simulink model "DC_Charger"  (R2024b)
settings: Solver=ode23t  StartTime=0.0  StopTime=inf  FixedStep=1e-6  MaxStep=1/(5*inverter.SwitchFrequency)  RelTol=1e-3  AbsTol=1e-3
undefined symbols (not defined in the file or in its folder): battery, inverter, rectifier
libraries: nesl_utility x38, fl_lib x26, ee_lib x14, batteryecm_lib x3, eePwmGenerator x2, eeTransforms x2, eeSinusoidalMeasurement x1, slpidlib x1, eePwmGeneratorThreeLevel x1, eePwmGeneratorTwoLevel x1, simulink_extras x1
(part 3 of 3)

== system DC_Charger/EV Battery/i ==
  Current Sensor : fl_lib/Electrical/Electrical Sensors/Current Sensor
  PS-Simulink Converter1 : nesl_utility/PS-Simulink Converter  PhysicalDomain=network_engine_domain  SubClassName=ps_output  LeftPortType=input  RightPortType=output  PseudoPeriodic=off  Frequencies=[]  VectorFormat=1-D array  Unit=1  AffineConversion=off
  Rate Transition : RateTransition  OutPortSampleTime=1/(10*inverter.SwitchFrequency)
  + : PMIOPort  Side=Left
  - : PMIOPort  Port=2  Side=Right
  I : Outport
  wires:
  Rate Transition/1 -> I/1
  PS-Simulink Converter1/1 -> Rate Transition/1
  connections:
  Current Sensor/RConn1 -- PS-Simulink Converter1/LConn1
  Current Sensor/RConn2 -- -/RConn1
  Current Sensor/LConn1 -- +/RConn1

== system DC_Charger/EV Battery/v ==
  PS-Simulink Converter : nesl_utility/PS-Simulink Converter  PhysicalDomain=network_engine_domain  SubClassName=ps_output  LeftPortType=input  RightPortType=output  PseudoPeriodic=off  Frequencies=[]  VectorFormat=1-D array  Unit=1  AffineConversion=off
  Rate Transition : RateTransition  OutPortSampleTime=1/(10*inverter.SwitchFrequency)
  Voltage Sensor : fl_lib/Electrical/Electrical Sensors/Voltage Sensor
  + : PMIOPort  Side=Right
  - : PMIOPort  Port=2  Side=Left
  V : Outport
  wires:
  PS-Simulink Converter/1 -> Rate Transition/1
  Rate Transition/1 -> V/1
  connections:
  +/RConn1 -- Voltage Sensor/LConn1
  -/RConn1 -- Voltage Sensor/RConn2
  Voltage Sensor/RConn1 -- PS-Simulink Converter/LConn1

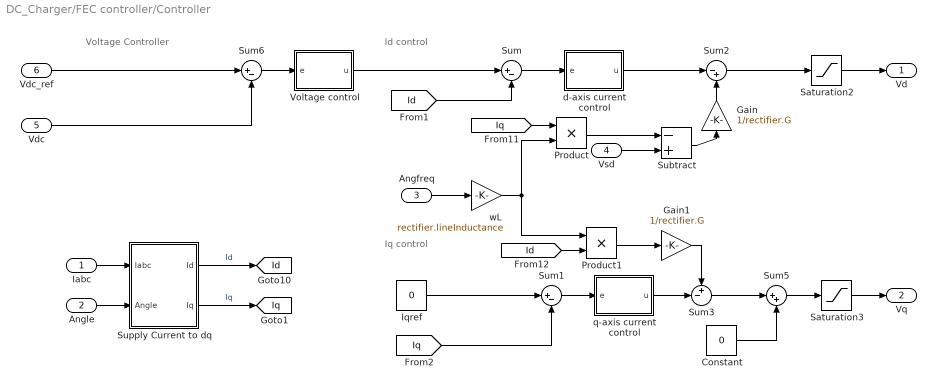
== system DC_Charger/FEC controller/Controller ==
  note: Id control
  note: Voltage Controller
  note: Iq control
  Iabc : Inport
  Angle : Inport  Port=2
  Angfreq : Inport  Port=3
  Vsd : Inport  Port=4
  Vdc : Inport  Port=5
  Vdc_ref : Inport  Port=6
  Constant : Constant  Value=0
  Gain : Gain  Gain=1/rectifier.G
  Gain1 : Gain  Gain=1/rectifier.G
  Iqref : Constant  Value=0
  Product : Product
  Product1 : Product
  Saturation2 : Saturate  UpperLimit=4  LowerLimit=-3
  Saturation3 : Saturate  UpperLimit=1  LowerLimit=-1
  Subtract : Sum  Inputs=-+
  Sum : Sum  Inputs=|+-
  Sum1 : Sum  Inputs=|+-
  Sum2 : Sum  Inputs=|-+
  Sum3 : Sum  Inputs=+-|
  Sum5 : Sum  Inputs=|++
  Sum6 : Sum  Inputs=|+-
  Supply Current to dq : Subsystem
  Voltage control : Subsystem
  d-axis current control : Subsystem
  q-axis current control : Subsystem
  wL : Gain  Gain=rectifier.lineInductance
  Vd : Outport  VectorParamsAs1DForOutWhenUnconnected=off
  Vq : Outport  Port=2  VectorParamsAs1DForOutWhenUnconnected=off
  tag scope: Id=global, Iq=global
  wires:
  Sum1/1 -> q-axis current control/1(e)
  wL/1 -> Product/2, Product1/1
  [Id] -> Product1/2
  [Iq] -> Product/1
  Sum3/1 -> Sum5/1
  Sum2/1 -> Saturation2/1
  Sum5/1 -> Saturation3/1
  Angfreq/1 -> wL/1
  Constant/1 -> Sum5/2
  Vdc/1 -> Sum6/2
  Sum/1 -> d-axis current control/1(e)
  [Id] -> Sum/2
  d-axis current control/1(u) -> Sum2/1
  q-axis current control/1(u) -> Sum3/2
  Supply Current to dq/1(Id) -> [Id]  "Id"
  Supply Current to dq/2(Iq) -> [Iq]  "Iq"
  Sum6/1 -> Voltage control/1(e)
  Saturation3/1 -> Vq/1
  Saturation2/1 -> Vd/1
  Iqref/1 -> Sum1/1
  [Iq] -> Sum1/2
  Voltage control/1(u) -> Sum/1
  Vdc_ref/1 -> Sum6/1
  Product1/1 -> Gain1/1
  Product/1 -> Subtract/1
  Vsd/1 -> Subtract/2
  Subtract/1 -> Gain/1
  Gain/1 -> Sum2/2
  Gain1/1 -> Sum3/1
  Iabc/1 -> Supply Current to dq/1(Iabc)
  Angle/1 -> Supply Current to dq/2(Angle)

== system DC_Charger/FEC controller/Modulation Signal ==
  Vd : Inport
  Vq : Inport  Port=2
  Angle : Inport  Port=3
  Constant : Constant  Value=0
  Gain : Gain  Gain=2/3
  Inverse Park Transform : eeTransforms/Inverse Park Transform  AxisAlignment=D-axis  PowerInvariant=off
  Mux1 : Mux  Inputs=3
  Saturation2 : Saturate  UpperLimit=1  LowerLimit=-1
  mabc : Outport  VectorParamsAs1DForOutWhenUnconnected=off
  wires:
  Gain/1 -> Saturation2/1
  Mux1/1 -> Inverse Park Transform/1
  Inverse Park Transform/1 -> Gain/1
  Constant/1 -> Mux1/3
  Vd/1 -> Mux1/1
  Vq/1 -> Mux1/2
  Angle/1 -> Inverse Park Transform/2
  Saturation2/1 -> mabc/1

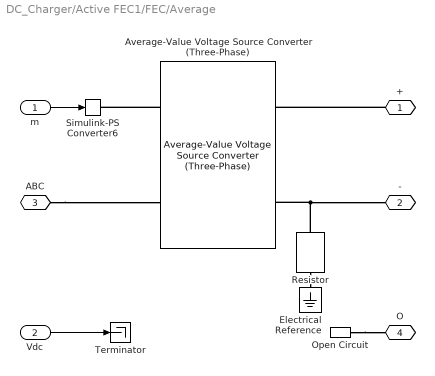
== system DC_Charger/Active FEC1/FEC/Average ==
  m : Inport
  Vdc : Inport  Port=2
  Average-Value Voltage Source Converter (Three-Phase) : ee_lib/Semiconductors & Converters/Converters/Average-Value Voltage Source Converter (Three-Phase)  port_option=ee.enum.threePhasePort.composite  frequency_option=ee.enum.converters.frequency.variable  input_option=ee.enum.converters.inputOption.ModWave  FRated=60 Hz  losses_parameterization=ee.enum.converters.losses.fixed  Pfixed=1 W  ks=0.01  kc1=1.7 V  kc2=0.01 Ohm  Ploss_vect=[100, 800, 1870, 3250, 4900] W  Irms_vect=[10, 100, 200, 300, 400] A  Vdc_nom=300 V  thermal_mass=30000 J/K  temperature_specify=off  temperature_priority=High  temperature=298.15 K  temperature_nominal_specify=off  temperature_nominal_value=1  temperature_nominal_unit=K
      settings: InternalSimscapePortConfiguration="{\"Bottom\":[],\"Left\":[{\"id\":\"ModWave\",\"label\":\"ModWave\",\"type\":\"input\"},{\"id\":\"N\",\"label\":\"~\",\"type\":\"foundation.electrical.three_phase\"}],\"Right\":[{\"id\":\"p\",\"label\":\"+\",\"type\":\"foundation.electrical.electrical\"},{\"id\":\"n\",\"label\":\"-\",\"type\":\"foundation.electrical.electrical\"}],\"Top\":[]}"
  Electrical Reference : fl_lib/Electrical/Electrical Elements/Electrical Reference
  Open Circuit : fl_lib/Electrical/Electrical Elements/Open Circuit  v_specify=off  v_priority=None  v=0 V  v_nominal_specify=off  v_nominal_value=1  v_nominal_unit=V
  Resistor : fl_lib/Electrical/Electrical Elements/Resistor  R=1e6 Ohm  i_specify=off  i_priority=None  i=0 A  i_nominal_specify=off  i_nominal_value=1  i_nominal_unit=A  v_specify=off  v_priority=None  v=0 V  v_nominal_specify=off  v_nominal_value=1  v_nominal_unit=V
  Simulink-PS Converter6 : nesl_utility/Simulink-PS Converter  PhysicalDomain=network_engine_domain  SubClassName=ps_input  LeftPortType=input  RightPortType=output  PseudoPeriodic=off  Frequencies=[]  NoiseDistribution=none  NoiseParameters=[]  Unit=1  AffineConversion=off  FilteringAndDerivatives=provide  SimscapeFilterOrder=1  InputFilterTimeConstant=0.001  UdotUserProvided=0
  Terminator : Terminator
  + : PMIOPort  Side=Right
  - : PMIOPort  Port=2  Side=Right
  ABC : PMIOPort  Port=3  Side=Left
  O : PMIOPort  Port=4  Side=Right
  wires:
  m/1 -> Simulink-PS Converter6/1
  Vdc/1 -> Terminator/1
  connections:
  Open Circuit/LConn1 -- O/RConn1
  Average-Value Voltage Source Converter (Three-Phase)/LConn1 -- Simulink-PS Converter6/RConn1
  ABC/RConn1 -- Average-Value Voltage Source Converter (Three-Phase)/LConn2
  +/RConn1 -- Average-Value Voltage Source Converter (Three-Phase)/RConn1
  Resistor/LConn1 -- Average-Value Voltage Source Converter (Three-Phase)/RConn2 -- -/RConn1
  Resistor/RConn1 -- Electrical Reference/LConn1

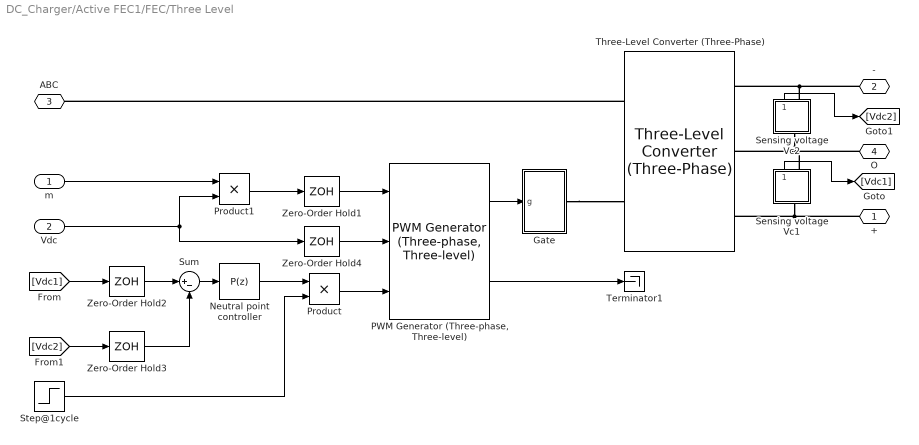
== system DC_Charger/Active FEC1/FEC/Three Level ==
  m : Inport
  Vdc : Inport  Port=2
  Gate : Subsystem
  Neutral point controller : slpidlib/PID Controller  Controller=P  Form=Parallel  TimeDomain=Discrete-time  UseExternalTs=off  SampleTime=-1  IntegratorMethod=Forward Euler  FilterMethod=Forward Euler  ControllerParametersSource=internal  P=0.001  I=80/2  UseKiTs=off  D=0  UseExternalDerivativeSource=off  N=100  UseFilter=on  TunerSelectOption=Transfer Function Based (PID Tuner App)  ZeroCross=off  InitialConditionSource=internal  InitialConditionForIntegrator=0  InitialConditionForFilter=0  DifferentiatorICPrevScaledInput=0  ExternalReset=none  TrackingMode=off  Kt=1  LimitOutput=on  SatLimitsSource=internal  UpperSaturationLimit=1  LowerSaturationLimit=-1  LinearizeAsGain=on  AntiWindupMode=back-calculation  Kb=1000  LimitIntegrator=off  UpperIntegratorSaturationLimit=inf  LowerIntegratorSaturationLimit=-inf  POutMin=[]  POutMax=[]  IOutMin=[]  IOutMax=[]  DOutMin=[]  DOutMax=[]  NOutMin=[]  NOutMax=[]  SumOutMin=[]  SumOutMax=[]  SaturationOutMin=[]  SaturationOutMax=[]  PParamMin=[]  PParamMax=[]  IParamMin=[]  IParamMax=[]  DParamMin=[]  DParamMax=[]  NParamMin=[]  NParamMax=[]  KbParamMin=[]  KbParamMax=[]  KtParamMin=[]  KtParamMax=[]  KbOutMin=[]  KbOutMax=[]  KtOutMin=[]  KtOutMax=[]  IntegratorOutMin=[]  IntegratorOutMax=[]  FilterOutMin=[]  FilterOutMax=[]  SumI1OutMin=[]  SumI1OutMax=[]  SumI2OutMin=[]  SumI2OutMax=[]  SumI3OutMin=[]  SumI3OutMax=[]  SumI4OutMin=[]  SumI4OutMax=[]  SumDOutMin=[]  SumDOutMax=[]  DifferentiatorOutMin=[]  DifferentiatorOutMax=[]  FilterDiffOutCoefMin=[]  FilterDiffOutCoefMax=[]  ReciprocalOutMin=[]  ReciprocalOutMax=[]  SumDenOutMin=[]  SumDenOutMax=[]  SumNumOutMin=[]  SumNumOutMax=[]  DivideOutMin=[]  DivideOutMax=[]  UdiffTsProdOutMin=[]  UdiffTsProdOutMax=[]  NTsProdOutMin=[]  NTsProdOutMax=[]  UintegralTsProdOutMin=[]  UintegralTsProdOutMax=[]  UngainTsProdOutMin=[]  UngainTsProdOutMax=[]  ClampingZeroOutDataTypeStr=Inherit: Inherit via back propagation  ClampingZeroOutMin=[]  ClampingZeroOutMax=[]  FilterDenConstantOutDataTypeStr=Inherit: Inherit via back propagation  FilterDenConstantOutMin=[]  FilterDenConstantOutMax=[]  PCopyOutDataTypeStr=Inherit: Inherit via back propagation  PCopyOutMin=[]  PCopyOutMax=[]  NCopyOutDataTypeStr=Inherit: Inherit via back propagation  NCopyOutMin=[]  NCopyOutMax=[]  IntegratorContinuousStateAttributes=''  IntegratorStateMustResolveToSignalObject=off  IntegratorRTWStateStorageClass=Auto  FilterContinuousStateAttributes=''  FilterStateMustResolveToSignalObject=off  FilterRTWStateStorageClass=Auto  ParallelPVariant=InternalParameters  IdealPVariant=Disabled  IVariant=Disabled  DVariant=Disabled  IntegratorVariant=Disabled  SatVariant=Enabled  AWVariant=Disabled  PCopyVariant=Disabled  TRVariant=Disabled  FdbkBlocksVariant=Forward  IdealPFdbkVariant=Disabled  SatFdbkVariant=Disabled  DerivativeFilterVariant=Disabled  NVariant=Disabled  NCopyVariant=Disabled_SignalSpec  FilterICVariant=Disabled  IntegratorICVariant=Disabled  ExternalResetVariant=Disabled  TRSumVariant=Passthrough  SumFdbkVariant=Disabled  SumVariant=Passthrough_P  TsampFilterVariant=InternalTs  TsampNgainVariant=Passthrough  TsampIntegralVariant=Disabled_SignalSpec  ExternalSaturationOutDataTypeStr=Inherit: Same as second input  DerivativeSourceVariant=Disabled  PreIntVariant=InternalPreInt
  "PWM Generator (Three-phase, Three-level)" : eePwmGeneratorThreeLevel/PWM Generator (Three-phase, Three-level)  CPWMMode=SPWM: sinusoidal PWM  fsw=rectifier.SwitchFrequency  Ts=1/(10*rectifier.SwitchFrequency)
      settings: SamplingMode=Natural
  Product : Product
  Product1 : Product
  Sensing voltage Vc1 : Subsystem
      mask Display: disp('Vdc1')
  Sensing voltage Vc2 : Subsystem
      mask Display: disp('Vdc2')
  Step@1cycle : Step  Time=1/rectifier.SystemFrequency  SampleTime=1/(10*rectifier.SwitchFrequency)
  Sum : Sum  Inputs=|+-
  Terminator1 : Terminator
  Three-Level Converter (Three-Phase) : ee_lib/Semiconductors & Converters/Converters/Three-Level Converter (Three-Phase)  port_option=ee.enum.threePhasePort.composite  device_type=2  Vf=0.8 V  Ron=0.001 Ohm  Rds=0.001 Ohm  Goff=1e-6 1/Ohm  Vth=0.2 V  Vgt=1 V  Vgt_off=-1 V  Ih=1 A  K=0  diode_param=2  diode_Vf=0.8 V  diode_Ron=0.001 Ohm  diode_Goff=1e-5 1/Ohm  diode_C=50 nF  diode_iRM=-235 A  diode_iF=300 A  diode_idot=-50 A/us  diode_trr_param=1  diode_trr_factor=3  diode_trr=15 us  diode_Qrr=1500 s*uA  snubber_type=0  Cs=1e-7 F  Rs=0.1 Ohm
      settings: InternalSimscapePortConfiguration="{\"Bottom\":[],\"Left\":[{\"id\":\"G\",\"label\":\"G\",\"type\":\"foundation.electrical.twenty_four_phase\"},{\"id\":\"N\",\"label\":\"~\",\"type\":\"foundation.electrical.three_phase\"}],\"Right\":[{\"id\":\"p\",\"label\":\"+\",\"type\":\"foundation.electrical.electrical\"},{\"id\":\"z\",\"label\":\"0\",\"type\":\"foundation.electrical.electrical\"},{\"id\":\"n\",\"label\":\"-\",\"type\":\"foundation.electrical.electrical\"}],\"Top\":[]}"
  Zero-Order Hold1 : ZeroOrderHold  SampleTime=1/(10*rectifier.SwitchFrequency)
  Zero-Order Hold2 : ZeroOrderHold  SampleTime=1/(5*rectifier.SwitchFrequency)
  Zero-Order Hold3 : ZeroOrderHold  SampleTime=1/(5*rectifier.SwitchFrequency)
  Zero-Order Hold4 : ZeroOrderHold  SampleTime=1/(10*rectifier.SwitchFrequency)
  + : PMIOPort  Side=Right
  - : PMIOPort  Port=2  Side=Right
  ABC : PMIOPort  Port=3  Side=Left
  O : PMIOPort  Port=4  Side=Right
  wires:
  Sum/1 -> Neutral point controller/1
  Vdc/1 -> Zero-Order Hold4/1, Product1/2
  m/1 -> Product1/1
  Zero-Order Hold2/1 -> Sum/1
  Zero-Order Hold3/1 -> Sum/2
  Zero-Order Hold1/1 -> "PWM Generator (Three-phase, Three-level)"/1
  Zero-Order Hold4/1 -> "PWM Generator (Three-phase, Three-level)"/2
  "PWM Generator (Three-phase, Three-level)"/2 -> Terminator1/1
  Product1/1 -> Zero-Order Hold1/1
  [Vdc1] -> Zero-Order Hold2/1
  Step@1cycle/1 -> Product/2
  [Vdc2] -> Zero-Order Hold3/1
  Neutral point controller/1 -> Product/1
  Product/1 -> "PWM Generator (Three-phase, Three-level)"/3
  "PWM Generator (Three-phase, Three-level)"/1 -> Gate/1(g)
  Sensing voltage Vc1/1(Out1) -> [Vdc1]
  Sensing voltage Vc2/1(Out1) -> [Vdc2]
  connections:
  Sensing voltage Vc2/LConn1 -- Sensing voltage Vc1/RConn1 -- O/RConn1 -- Three-Level Converter (Three-Phase)/RConn2
  -/RConn1 -- Three-Level Converter (Three-Phase)/RConn3 -- Sensing voltage Vc2/RConn1
  +/RConn1 -- Three-Level Converter (Three-Phase)/RConn1 -- Sensing voltage Vc1/LConn1
  Three-Level Converter (Three-Phase)/LConn2 -- ABC/RConn1
  Gate/RConn1 -- Three-Level Converter (Three-Phase)/LConn1

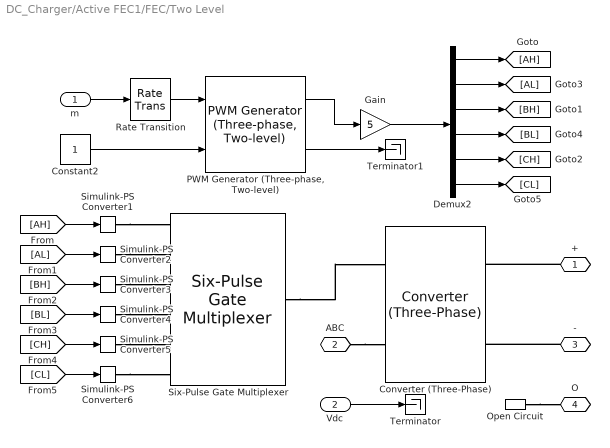
== system DC_Charger/Active FEC1/FEC/Two Level ==
  m : Inport
  Vdc : Inport  Port=2
  Constant2 : Constant
  Converter (Three-Phase) : ee_lib/Semiconductors & Converters/Converters/Converter (Three-Phase)  port_option=ee.enum.threePhasePort.composite  fidelity_option=ee.enum.converters.fidelity.detailed  device_type=ee.enum.converters.switchingdevice.ideal  showThermalPort=false  K=0  Vth=0.5 V  Vgt=1 V  Vgt_off=-1 V  Ih=1 A  Vf=0.8 V  Ron=0.001 Ohm  Rds=0.001 Ohm  Goff=1e-6 1/Ohm  Eon_scalar=22.86e-3 J  Eoff_scalar=17.14e-3 J  Eoff_natural_commutation=10e-3 J  Voff=300 V  Iout_scalar=600 A  onCurrentMeasDelay=0 s  useCurrentFromPreviousCycle=false  useVoltageFromPreviousCycle=false  diode_param=ee.enum.converters.protectiondiode.nodynamics  diode_Vf=0.06 V  diode_Ron=0.001 Ohm  diode_Goff=1e-5 1/Ohm  diode_C=50 nF  diode_iRM=-235 A  diode_iF=300 A  diode_idot=-50 A/us  diode_trr_param=ee.enum.converters.diodetrr.trr_factor  diode_trr_factor=3  diode_trr=15 us  diode_Qrr=1500 s*uA  diode_rec_loss_model=ee.enum.diode.reverseRecoveryModel.fixed  diode_ErecVal=0 J  diode_scaleWithIandV=false  diode_ErecMat=zeros(2, 3) J  diode_TjrecVec=[298.15, 398.15] K  diode_IfrecVec=[.1, 1, 10] A  diode_IrecVal=10 A  diode_VrecVal=10 V  diode_tFilter=1 / 1000 / 100 s  thermal_network_parameterization=ee.enum.thermalNetworkTopology.external  Rth=[.08, .5] K/W  Rth_Cauer=[.08, .1, .5] K/W  Rth_Foster=[.08, .14, .22, .16] K/W  thermal_mass_parameterization=ee.enum.thermalNetwork.timeconstant  thermal_mass=[.01, .5] J/K  thermal_mass_Cauer=[.01, .1, .5] J/K  thermal_mass_Foster=[.001, .005, .05, .5] J/K  thermal_time_constant=[.001, .2] s  thermal_time_constant_Cauer=[.001, .1, .2] s  thermal_time_constant_Foster=[7e-05, .0007, .01, .08] s  thermal_mass_initial_temperatures=[25, 25] degC  thermal_mass_initial_temperatures_Cauer=[25, 25, 25] degC  junction_thermal_mass=0.01 J/K  Tvec_initial_Foster=[25, 25, 25, 25] degC  snubber_type=ee.enum.converters.snubber.exclude  Cs=1e-7 F  Rs=0.1 Ohm  Vce_loss=[0, 150, 300] V
  Demux2 : Demux  Outputs=6
  Gain : Gain  Gain=5
  Open Circuit : fl_lib/Electrical/Electrical Elements/Open Circuit  v_specify=off  v_priority=None  v=0 V  v_nominal_specify=off  v_nominal_value=1  v_nominal_unit=V
  "PWM Generator (Three-phase, Two-level)" : eePwmGeneratorTwoLevel/PWM Generator (Three-phase, Two-level)  PWMMode=Continuous PWM (CPWM)  CPWMMode=SVM: space vector modulation  DPWMMode=60 DPWM: 60 degree discontinuous PWM  fsw=rectifier.SwitchFrequency  Ts=rectifier.VoltageSensorT
  Rate Transition : RateTransition  OutPortSampleTime=rectifier.VoltageSensorT
  Simulink-PS Converter{1..6} (6 alike) : nesl_utility/Simulink-PS Converter  PhysicalDomain=network_engine_domain  SubClassName=ps_input  LeftPortType=input  RightPortType=output  PseudoPeriodic=off  Frequencies=[]  NoiseDistribution=none  NoiseParameters=[]  Unit=1  AffineConversion=off  FilteringAndDerivatives=provide  SimscapeFilterOrder=1  InputFilterTimeConstant=0.001  UdotUserProvided=0
  Six-Pulse Gate Multiplexer : ee_lib/Semiconductors & Converters/Converters/Six-Pulse Gate Multiplexer  port_option=ee.enum.controlport.ps
  Terminator : Terminator
  Terminator1 : Terminator
  + : PMIOPort  Side=Right
  ABC : PMIOPort  Port=2  Side=Left
  - : PMIOPort  Port=3  Side=Right
  O : PMIOPort  Port=4  Side=Right
  wires:
  [AH] -> Simulink-PS Converter1/1
  [CL] -> Simulink-PS Converter6/1
  [AL] -> Simulink-PS Converter2/1
  [BL] -> Simulink-PS Converter4/1
  [CH] -> Simulink-PS Converter5/1
  [BH] -> Simulink-PS Converter3/1
  Gain/1 -> Demux2/1
  Rate Transition/1 -> "PWM Generator (Three-phase, Two-level)"/1
  Demux2/2 -> [AL]
  Demux2/1 -> [AH]
  Demux2/5 -> [CH]
  Demux2/3 -> [BH]
  "PWM Generator (Three-phase, Two-level)"/1 -> Gain/1
  Demux2/4 -> [BL]
  Demux2/6 -> [CL]
  Constant2/1 -> "PWM Generator (Three-phase, Two-level)"/2
  m/1 -> Rate Transition/1
  Vdc/1 -> Terminator/1
  "PWM Generator (Three-phase, Two-level)"/2 -> Terminator1/1
  connections:
  ABC/RConn1 -- Converter (Three-Phase)/LConn2
  Simulink-PS Converter1/RConn1 -- Six-Pulse Gate Multiplexer/LConn1
  Simulink-PS Converter2/RConn1 -- Six-Pulse Gate Multiplexer/LConn2
  Simulink-PS Converter3/RConn1 -- Six-Pulse Gate Multiplexer/LConn3
  Simulink-PS Converter4/RConn1 -- Six-Pulse Gate Multiplexer/LConn4
  Simulink-PS Converter5/RConn1 -- Six-Pulse Gate Multiplexer/LConn5
  Simulink-PS Converter6/RConn1 -- Six-Pulse Gate Multiplexer/LConn6
  Six-Pulse Gate Multiplexer/RConn1 -- Converter (Three-Phase)/LConn1
  +/RConn1 -- Converter (Three-Phase)/RConn1
  -/RConn1 -- Converter (Three-Phase)/RConn2
  Open Circuit/LConn1 -- O/RConn1

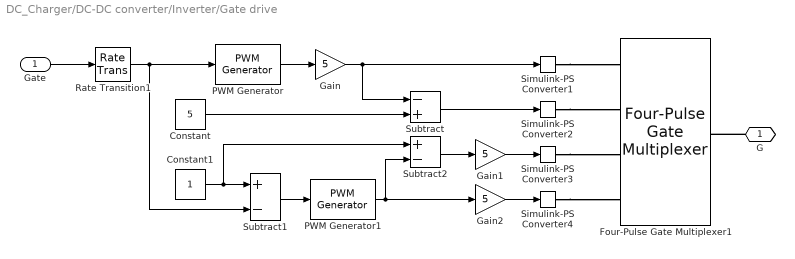
== system DC_Charger/DC-DC converter/Inverter/Gate drive ==
  Gate : Inport
  Constant : Constant  Value=5
  Constant1 : Constant
  Four-Pulse Gate Multiplexer1 : ee_lib/Semiconductors & Converters/Converters/Four-Pulse Gate Multiplexer  port_option=ee.enum.controlport.ps
      settings: InternalSimscapePortConfiguration="{\"Bottom\":[],\"Left\":[{\"id\":\"G1_ps\",\"label\":\"G1\",\"type\":\"input\"},{\"id\":\"G2_ps\",\"label\":\"G2\",\"type\":\"input\"},{\"id\":\"G3_ps\",\"label\":\"G3\",\"type\":\"input\"},{\"id\":\"G4_ps\",\"label\":\"G4\",\"type\":\"input\"}],\"Right\":[{\"id\":\"p\",\"label\":\"G\",\"type\":\"foundation.electrical.eight_phase\"}],\"Top\":[]}"
  Gain : Gain  Gain=5
  Gain1 : Gain  Gain=5
  Gain2 : Gain  Gain=5
  PWM Generator : eePwmGenerator/PWM Generator  CarrCount=Up  Tper=1/inverter.SwitchFrequency  Tdelay=0  Ts=1/(10*inverter.SwitchFrequency)
  PWM Generator1 : eePwmGenerator/PWM Generator  CarrCount=Up  Tper=1/inverter.SwitchFrequency  Tdelay=0  Ts=1/(10*inverter.SwitchFrequency)
  Rate Transition1 : RateTransition  OutPortSampleTime=1/(10*inverter.SwitchFrequency)
  Simulink-PS Converter{1..4} (4 alike) : nesl_utility/Simulink-PS Converter  PhysicalDomain=network_engine_domain  SubClassName=ps_input  LeftPortType=input  RightPortType=output  PseudoPeriodic=off  Frequencies=[]  NoiseDistribution=none  NoiseParameters=[]  Unit=1  AffineConversion=off  FilteringAndDerivatives=provide  SimscapeFilterOrder=1  InputFilterTimeConstant=0.001  UdotUserProvided=0
  Subtract : Sum  Inputs=-+
  Subtract1 : Sum  Inputs=+-
  Subtract2 : Sum  Inputs=+-
  G : PMIOPort  Side=Right
  wires:
  Rate Transition1/1 -> PWM Generator/1, Subtract1/2
  PWM Generator/1 -> Gain/1
  Constant/1 -> Subtract/2
  Gain/1 -> Simulink-PS Converter1/1, Subtract/1
  Subtract1/1 -> PWM Generator1/1
  PWM Generator1/1 -> Subtract2/2, Gain2/1
  Subtract/1 -> Simulink-PS Converter2/1
  Gain2/1 -> Simulink-PS Converter4/1
  Gate/1 -> Rate Transition1/1
  Subtract2/1 -> Gain1/1
  Gain1/1 -> Simulink-PS Converter3/1
  Constant1/1 -> Subtract2/1, Subtract1/1
  connections:
  G/RConn1 -- Four-Pulse Gate Multiplexer1/RConn1
  Simulink-PS Converter1/RConn1 -- Four-Pulse Gate Multiplexer1/LConn1
  Simulink-PS Converter2/RConn1 -- Four-Pulse Gate Multiplexer1/LConn2
  Simulink-PS Converter4/RConn1 -- Four-Pulse Gate Multiplexer1/LConn4
  Simulink-PS Converter3/RConn1 -- Four-Pulse Gate Multiplexer1/LConn3

== system DC_Charger/FEC controller/Controller/Supply Current to dq ==
  Iabc : Inport
  Angle : Inport  Port=2
  Demux : Demux  Outputs=3
  Gain1 : Gain  Gain=1.5
  Park Transform : eeTransforms/Park Transform  AxisAlignment=D-axis  PowerInvariant=off
  Terminator : Terminator
  Id : Outport  VectorParamsAs1DForOutWhenUnconnected=off
  Iq : Outport  Port=2  VectorParamsAs1DForOutWhenUnconnected=off
  wires:
  Demux/3 -> Terminator/1
  Gain1/1 -> Demux/1
  Park Transform/1 -> Gain1/1
  Demux/2 -> Iq/1
  Demux/1 -> Id/1
  Iabc/1 -> Park Transform/1
  Angle/1 -> Park Transform/2

== system DC_Charger/FEC controller/Controller/Voltage control ==
  e : Inport
  Integrator : Integrator  LimitOutput=on  UpperSaturationLimit=500  LowerSaturationLimit=-500
  Ki : Gain  Gain=1/rectifier.controller.VoltageT
  Kp : Gain  Gain=rectifier.controller.VoltageG
  Saturation : Saturate  UpperLimit=600  LowerLimit=-600
  Sum7 : Sum  Inputs=|++
  u : Outport  VectorParamsAs1DForOutWhenUnconnected=off
  wires:
  Integrator/1 -> Sum7/2
  Sum7/1 -> Saturation/1
  e/1 -> Kp/1
  Kp/1 -> Ki/1, Sum7/1
  Ki/1 -> Integrator/1
  Saturation/1 -> u/1

== system DC_Charger/FEC controller/Controller/d-axis current control ==
  e : Inport
  Integrator : Integrator  LimitOutput=on  UpperSaturationLimit=10  LowerSaturationLimit=-10
  Ki : Gain  Gain=1/rectifier.controller.CurrentT
  Kp : Gain  Gain=rectifier.controller.CurrentG
  Saturation : Saturate  UpperLimit=4  LowerLimit=-4
  Sum7 : Sum  Inputs=|++
  u : Outport  VectorParamsAs1DForOutWhenUnconnected=off
  wires:
  Integrator/1 -> Sum7/2
  Sum7/1 -> Saturation/1
  e/1 -> Kp/1
  Kp/1 -> Ki/1, Sum7/1
  Ki/1 -> Integrator/1
  Saturation/1 -> u/1

== system DC_Charger/FEC controller/Controller/q-axis current control ==
  e : Inport
  Integrator : Integrator  LimitOutput=on  UpperSaturationLimit=8  LowerSaturationLimit=-8
  Ki : Gain  Gain=1/rectifier.controller.CurrentT
  Kp : Gain  Gain=rectifier.controller.CurrentG
  Saturation : Saturate  UpperLimit=3  LowerLimit=-3
  Sum7 : Sum  Inputs=|++
  u : Outport  VectorParamsAs1DForOutWhenUnconnected=off
  wires:
  Ki/1 -> Integrator/1
  Kp/1 -> Sum7/1, Ki/1
  e/1 -> Kp/1
  Sum7/1 -> Saturation/1
  Saturation/1 -> u/1
  Integrator/1 -> Sum7/2

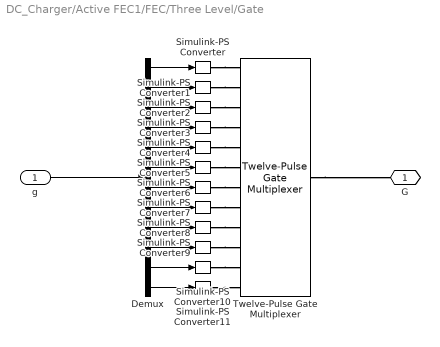
== system DC_Charger/Active FEC1/FEC/Three Level/Gate ==
  g : Inport
  Demux : Demux  Outputs=12
  Simulink-PS Converter{,1..11} (12 alike) : nesl_utility/Simulink-PS Converter  PhysicalDomain=network_engine_domain  SubClassName=ps_input  LeftPortType=input  RightPortType=output  PseudoPeriodic=off  Frequencies=[]  NoiseDistribution=none  NoiseParameters=[]  Unit=1  AffineConversion=off  FilteringAndDerivatives=zero  SimscapeFilterOrder=1  InputFilterTimeConstant=0.001  UdotUserProvided=1
  Twelve-Pulse Gate Multiplexer : ee_lib/Semiconductors & Converters/Converters/Twelve-Pulse Gate Multiplexer  port_option=ee.enum.controlport.ps
      settings: InternalSimscapePortConfiguration="{\"Bottom\":[],\"Left\":[{\"id\":\"Ga1_ps\",\"label\":\"Ga(1)\",\"type\":\"input\"},{\"id\":\"Ga2_ps\",\"label\":\"Ga(2)\",\"type\":\"input\"},{\"id\":\"Ga3_ps\",\"label\":\"Ga(3)\",\"type\":\"input\"},{\"id\":\"Ga4_ps\",\"label\":\"Ga(4)\",\"type\":\"input\"},{\"id\":\"Gb1_ps\",\"label\":\"Gb(1)\",\"type\":\"input\"},{\"id\":\"Gb2_ps\",\"label\":\"Gb(2)\",\"type\":\"input\"},{\"id\":\"Gb3_ps\",\"label\":\"Gb(3)\",\"type\":\"input\"},{\"id\":\"Gb4_ps\",\"label\":\"Gb(4)\",\"type\":\"input\"},{\"id\":\"Gc1_ps\",\"label\":\"Gc(1)\",\"type\":\"input\"},{\"id\":\"Gc2_ps\",\"label\":\"Gc(2)\",\"type\":\"input\"},{\"id\":\"Gc3_ps\",\"label\":\"Gc(3)\",\"type\":\"input\"},{\"id\":\"Gc4_ps\",\"label\":\"Gc(4)\",\"type\":\"input\"}],\"Right\":[{\"id\":\"p\",\"label\":\"G\",\"type\":\"foundation.electrical.twenty_four_phase\"}],\"Top\":[]}"
  G : PMIOPort  Side=Right
  wires:
  g/1 -> Demux/1
  Demux/5 -> Simulink-PS Converter4/1
  Demux/10 -> Simulink-PS Converter9/1
  Demux/2 -> Simulink-PS Converter1/1
  Demux/9 -> Simulink-PS Converter8/1
  Demux/12 -> Simulink-PS Converter11/1
  Demux/3 -> Simulink-PS Converter2/1
  Demux/7 -> Simulink-PS Converter6/1
  Demux/6 -> Simulink-PS Converter5/1
  Demux/4 -> Simulink-PS Converter3/1
  Demux/1 -> Simulink-PS Converter/1
  Demux/11 -> Simulink-PS Converter10/1
  Demux/8 -> Simulink-PS Converter7/1
  connections:
  Simulink-PS Converter10/RConn1 -- Twelve-Pulse Gate Multiplexer/LConn11
  Simulink-PS Converter8/RConn1 -- Twelve-Pulse Gate Multiplexer/LConn9
  Simulink-PS Converter/RConn1 -- Twelve-Pulse Gate Multiplexer/LConn1
  Simulink-PS Converter11/RConn1 -- Twelve-Pulse Gate Multiplexer/LConn12
  Simulink-PS Converter3/RConn1 -- Twelve-Pulse Gate Multiplexer/LConn4
  Simulink-PS Converter2/RConn1 -- Twelve-Pulse Gate Multiplexer/LConn3
  Simulink-PS Converter4/RConn1 -- Twelve-Pulse Gate Multiplexer/LConn5
  Simulink-PS Converter1/RConn1 -- Twelve-Pulse Gate Multiplexer/LConn2
  Twelve-Pulse Gate Multiplexer/RConn1 -- G/RConn1
  Simulink-PS Converter5/RConn1 -- Twelve-Pulse Gate Multiplexer/LConn6
  Simulink-PS Converter9/RConn1 -- Twelve-Pulse Gate Multiplexer/LConn10
  Simulink-PS Converter6/RConn1 -- Twelve-Pulse Gate Multiplexer/LConn7
  Simulink-PS Converter7/RConn1 -- Twelve-Pulse Gate Multiplexer/LConn8

== system DC_Charger/Active FEC1/FEC/Three Level/Sensing voltage Vc1 ==
  PS-Simulink Converter : nesl_utility/PS-Simulink Converter  PhysicalDomain=network_engine_domain  SubClassName=ps_output  LeftPortType=input  RightPortType=output  PseudoPeriodic=off  Frequencies=[]  VectorFormat=1-D array  Unit=1  AffineConversion=off
  Sensor dynamics : TransferFcn  Numerator=rectifier.VoltageSensorG  Denominator=[rectifier.VoltageSensorT 1]
  Vc1 : fl_lib/Electrical/Electrical Sensors/Voltage Sensor
  + : PMIOPort  Side=Left
  - : PMIOPort  Port=2  Side=Right
  Out1 : Outport
  wires:
  PS-Simulink Converter/1 -> Sensor dynamics/1
  Sensor dynamics/1 -> Out1/1
  connections:
  Vc1/RConn2 -- -/RConn1
  Vc1/LConn1 -- +/RConn1
  PS-Simulink Converter/LConn1 -- Vc1/RConn1

== system DC_Charger/Active FEC1/FEC/Three Level/Sensing voltage Vc2 ==
  PS-Simulink Converter : nesl_utility/PS-Simulink Converter  PhysicalDomain=network_engine_domain  SubClassName=ps_output  LeftPortType=input  RightPortType=output  PseudoPeriodic=off  Frequencies=[]  VectorFormat=1-D array  Unit=1  AffineConversion=off
  Sensor dynamics : TransferFcn  Numerator=rectifier.VoltageSensorG  Denominator=[rectifier.VoltageSensorT 1]
  Vc2 : fl_lib/Electrical/Electrical Sensors/Voltage Sensor
  Conn1 : PMIOPort  Side=Left
  Conn3 : PMIOPort  Port=2  Side=Right
  Out1 : Outport
  wires:
  Sensor dynamics/1 -> Out1/1
  PS-Simulink Converter/1 -> Sensor dynamics/1
  connections:
  Vc2/RConn2 -- Conn3/RConn1
  Vc2/LConn1 -- Conn1/RConn1
  PS-Simulink Converter/LConn1 -- Vc2/RConn1
